simulink model "thirdmodel"  (R2021b)
settings: Solver=VariableStepAuto  StartTime=0.0  StopTime=100  RelTol=1e-3
undefined symbols (not defined in the file): kr, Td, Ti, Tp
settings Model: Creator=Chyba Ja  LastModifiedBy=Chyba Ja

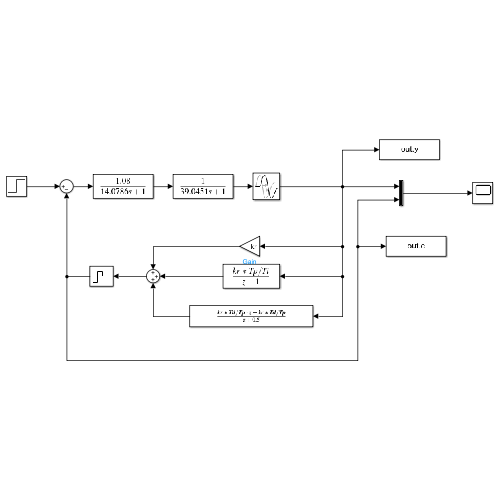
[thumbnail: Simulink's stored preview of the top-level diagram]
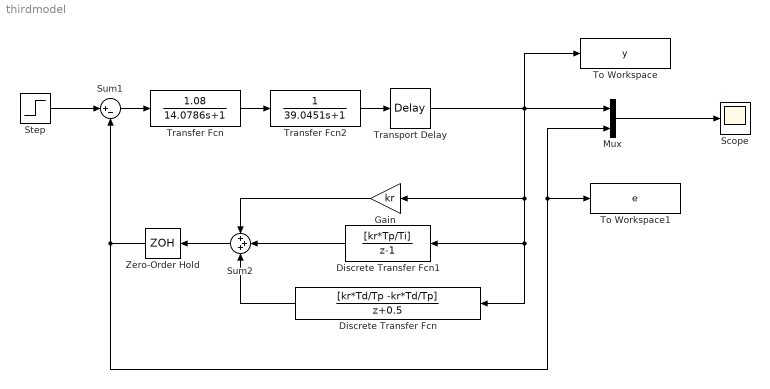
== system thirdmodel ==
  Discrete Transfer Fcn : DiscreteTransferFcn  Numerator=[kr*Td/Tp -kr*Td/Tp]
  Discrete Transfer Fcn1 : DiscreteTransferFcn  Numerator=[kr*Tp/Ti]  Denominator=[1 -1]
  Gain : Gain  Gain=kr
  Mux : Mux  Inputs=2
  Scope : Scope
  Step : Step  SampleTime=0
  Sum1 : Sum  Inputs=|+-
  Sum2 : Sum  Inputs=+++
  To Workspace : ToWorkspace  VariableName=y  SaveFormat=Timeseries  SampleTime=-1
  To Workspace1 : ToWorkspace  VariableName=e  SaveFormat=Timeseries  SampleTime=-1
  Transfer Fcn : TransferFcn  Numerator=[1.08]  Denominator=[14.0786 1]
  Transfer Fcn2 : TransferFcn  Denominator=[39.0451 1]
  Transport Delay : TransportDelay  DelayTime=15.1975
  Zero-Order Hold : ZeroOrderHold  SampleTime=Tp
  wires:
  Mux/1 -> Scope/1
  Sum1/1 -> Transfer Fcn/1
  Step/1 -> Sum1/1
  Sum2/1 -> Zero-Order Hold/1
  Gain/1 -> Sum2/1
  Discrete Transfer Fcn/1 -> Sum2/3
  Discrete Transfer Fcn1/1 -> Sum2/2
  Transport Delay/1 -> To Workspace/1, Discrete Transfer Fcn1/1, Discrete Transfer Fcn/1, Gain/1, Mux/1
  Transfer Fcn/1 -> Transfer Fcn2/1
  Transfer Fcn2/1 -> Transport Delay/1
  Zero-Order Hold/1 -> Sum1/2, To Workspace1/1, Mux/2
